simulink model "Wind_Turbine"  (Simulink 7.9)
settings: Solver=ode23t  StartTime=0.0  StopTime=80  MaxStep=0.01  RelTol=1e-5  AbsTol=1e-4
PreLoadFcn:
  | warning off Simulink:Commands:LoadMdlParameterizedLink
PostLoadFcn:
  | warning off Simulink:blocks:MatchingGotoNotFound
  | warning off Simulink:blocks:MatchingFromNotFound
  | warning('off','Simulink:SL_OutputNotConnected');
  | warning off Simulink:Engine:SaveWithParameterizedLinks_Warning
  | warning off Simulink:Engine:SaveWithDisabledLinks_Warning
  | warning('off','Simulink:fixpoint:fxpParameterPrecisionLoss');
  | warning off Simulink:blocks:DTConversionUncessary
  | warning off ne_sli:simulator:input:FilteredInputs
  | 
  | Setup_WT_Configurations
StartFcn:
  | tic
StopFcn:
  | Elapsed_Sim_Time = toc;
  | disp(['Elapsed time is ' num2str(Elapsed_Sim_Time)]);
undefined symbols (not defined in the file or in its folder): radps2rpm, WT_Params
libraries: powerlib x6, Wind_Lib x1, Blades_Lib x1, Generator_Lib x1, mblibv1 x1, Main_Controller_Lib x1, Nacelle_Lib x1, Pitch_Controller_Lib x1, Tower x1, Turbine_Input_Lib x1, Yaw_Controller_Lib x1
Description:
  | Copyright 2011 MathWorks, Inc.
settings Model: Creator=smiller  LastModifiedBy=smiller
settings SolverCC: MaxConsecutiveMinStep=5
settings DataIOCC: SaveFinalState=on
settings DebuggingCC: AlgebraicLoopMsg=error  ArtificialAlgebraicLoopMsg=none  SolverPrmCheckMsg=none  Int32ToFloatConvMsg=none  UnnecessaryDatatypeConvMsg=warning  FcnCallInpInsideContextMsg=Use local settings  StrictBusMsg=Warning
settings HardwareCC: TargetEndianess=LittleEndian  TargetHWDeviceType=MATLAB Host  ProdEqTarget=off
settings SFSimCC: SimParseCustomCode=off
settings RTWCC: ProcessScript=grt_make_rtw_hook
settings GRTTargetCC: CombineOutputUpdateFcns=off  GRTInterface=on
settings SimMechanicsCC: VisOnUpdateDiagram=on  VisDuringSimulation=on  FramesToBeSkipped=5  AnimationDelay=0  LastVizWinPosition=[16 233 560 424]  CamPosition=[-49.333;156.594;63.1057;]  CamTarget=[-1.98114;98.9678;-2.9194;]  CamUpVector=[0.335262;0.815674;-0.471461;]  CamHeight=16.8988  VisBackgroundColor=[0.678431;0.921569;1;]  DefaultBodyColor=[1;0;0;]
settings ConfigurationSet: Description=SimMechanics 2G

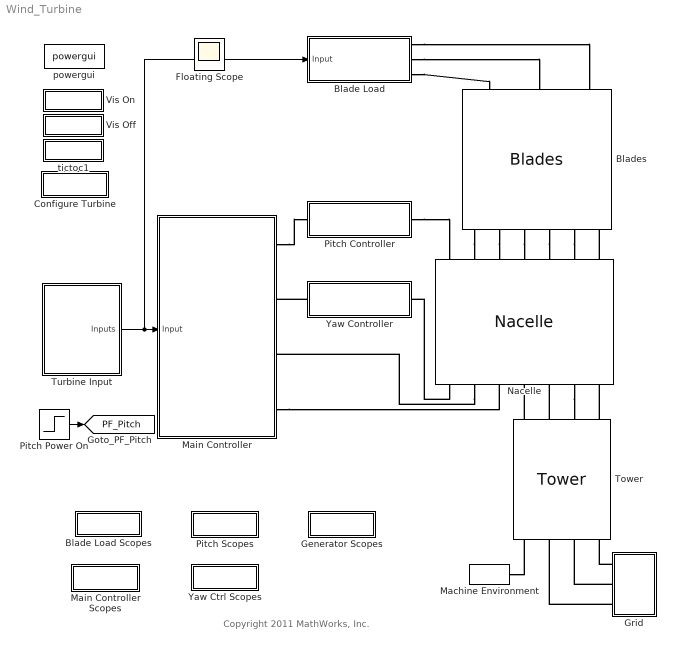
== system Wind_Turbine ==
  note: Copyright 2011 MathWorks, Inc.
  Blade Load : Subsystem  BlockChoice=Lift and Drag
      settings: AttributesFormatString=%<BlockChoice>  TemplateBlock=Wind_Lib/Blade Load  MemberBlocks=Lift and Drag,Lift and Drag (Simscape),Segments,Torque
  Blade Load Scopes : Subsystem  AncestorBlock=Wind_Lib/Blade Load Scopes
  Blades : Blades_Lib/Blades  RequirementInfo={'other' 'Wind_Turbine_Requirements.doc' '@overall_system' 'true' 'Blade Requirements ' ' ' } %GIDa_31eb547b_9de2_416c_ba1a_e68e51a35149  SystemSampleTime=-1
  Configure Turbine : Subsystem
  Generator Scopes : Subsystem  AncestorBlock=Generator_Lib/Generator Scopes
  Grid : Subsystem
  Machine Environment : mblibv1/Bodies/Machine Environment  PortType=env  PhysicalDomain=Mechanical  DialogTemplateClass=MECH.MachineEnvironment  SyncWhenCopied=off  Gravity=[0 -9.81 0]*0  GravityUnits=m/s^2  GravityAsSignal=off  Dimensionality=Auto-detect  AnalysisType=Forward dynamics  LinearAssemblyTolerance=1e-3  LinearAssemblyToleranceUnits=m  AngularAssemblyTolerance=1e-3  AngularAssemblyToleranceUnits=rad  ConstraintSolverType=Machine precision  ConstraintRelTolerance=1e-4  ConstraintAbsTolerance=1e-4  UseRobustSingularityHandling=off  RedundancyAnalysisToleranceType=Automatically select tolerance  RedundancyAnalysisTolerance=1e-14  StatePerturbationType=Fixed  PerturbationSize=1e-5  VisualizeMachine=on  BodyVisualizationType=Use model default body geometries  BodyColorSelMode=Use model default  DefaultBodyColor=[1 0 0]
  Main Controller : Subsystem  BlockChoice=Wind Input
      settings: AttributesFormatString=%<BlockChoice>  TemplateBlock=Main_Controller_Lib/Main Controller  MemberBlocks=Direct Input,Wind Input
  Main Controller Scopes : Subsystem  AncestorBlock=Main_Controller_Lib/Main Controller Scopes
  Nacelle : Nacelle_Lib/Nacelle  SystemSampleTime=-1
      link override Geartrain: BlockChoice=Empty
      link override Generator: BlockChoice=Simple
      link override Generator/Full/B_Gen/Model/VI/Ia: GotoTag=LibraryTag_Ia
      link override Generator/Full/B_Gen/Model/VI/Ib: GotoTag=LibraryTag_Ib
      link override Generator/Full/B_Gen/Model/VI/Ic: GotoTag=LibraryTag_Ic
      link override Generator/Full/B_Gen/Model/VI/Va: GotoTag=LibraryTag_Va
      link override Generator/Full/B_Gen/Model/VI/Vb: GotoTag=LibraryTag_Vb
      link override Generator/Full/B_Gen/Model/VI/Vc: GotoTag=LibraryTag_Vc
      link override Hub Axis: BlockChoice=Rotate
      link override Hub Axis/Rotate/3D-1D Mechanical Interface/Revolute - Rotational Interface/Joint Actuator: Primitive=R1  ActuationStyle=Force  TorqueUnits=N*m
      link override Hub Axis/Rotate/3D-1D Mechanical Interface/Revolute - Rotational Interface/Joint Sensor: Primitive=R1  Angle=off  ArcVelocity=on  ArcVelocityUnits=rad/s  ArcAcceleration=off  CoordPosition=off  Velocity=off  Acceleration=off  Quaternion=off  QuaternionDT=off  QuaternionDDT=off  Force=off  Torque=off  ReactionForce=off  ReactionMoment=off
      link override Hub Axis/Rotate/3D-1D Mechanical Interface/Revolute - Rotational Interface/PS-Simulink Converter: Unit=N*m
      link override Hub Axis/Rotate/3D-1D Mechanical Interface/Revolute - Rotational Interface/Simulink-PS Converter: Unit=rad/s
      link override Pitch System: BlockChoice=Ideal
      link override Yaw System: BlockChoice=Ideal Actuator
  Pitch Controller : Subsystem  BlockChoice=PI on AoA
      link override PI on AoA/Pitch Controller/Determine Pitch Command/Determine Angle of Attack if Pitch Angle Were 0/radps2mps: Gain=WT_Params.Blade.length
      settings: AttributesFormatString=%<BlockChoice>  TemplateBlock=Pitch_Controller_Lib/Pitch Controller  MemberBlocks=Inner Loop,PI on AoA
  Pitch Power On : Step  Time=20  Before=24  After=24  SampleTime=0
  Pitch Scopes : Subsystem  AncestorBlock=Pitch_Controller_Lib/Pitch Scopes
  Tower : Tower/Tower  RequirementInfo={'other' 'Wind_Turbine_Requirements.doc' '@Simulink_requirement_item_8' 'true' 'Tower Requirements' '' } %GIDa_4943b1c2_7ab1_472c_939d_e8be874b5a74  SystemSampleTime=-1
  Turbine Input : Subsystem  BlockChoice=Wind
      settings: AttributesFormatString=%<BlockChoice>  TemplateBlock=Turbine_Input_Lib/Turbine Input  MemberBlocks=Commands,Wind,Wind Cut Out,Wind High Speed,Wind Vary Speed
  Vis Off : Subsystem
      settings: OpenFcn=|
      | Temp_ENVHa= get_param(find_system(gcs,'LookUnderMasks','all','FollowLinks','on','ClassName','Environment'),'handle');
      | 
      | set_param(Temp_ENVHa{1},'VisualizeMachine','off');
      | 
      | set_param(gcs,'VisDuringSimulation','off')
      | set_param(gcs,'VisOnUpdateDiagram','off')
      mask Display: disp('Vis Off')
  Vis On : Subsystem
      settings: OpenFcn=|
      | Temp_ENVHa= get_param(find_system(gcs,'LookUnderMasks','all','FollowLinks','on','ClassName','Environment'),'handle');
      | 
      | set_param(Temp_ENVHa{1},'VisualizeMachine','on');
      | clear Temp_ENVHa;
      | set_param(gcs,'VisDuringSimulation','on')
      | set_param(gcs,'VisOnUpdateDiagram','on')
      mask Display: disp('Vis On')
  Yaw Controller : Subsystem  RequirementInfo={'other' 'Wind_Turbine_Requirements.doc' '@Simulink_requirement_item_7' 'true' 'Yaw Controller Requirements' '' } %GIDa_4e251ab5_598c_48b3_adbc_649df3f133e8  BlockChoice=Speed Limit
      settings: AttributesFormatString=%<BlockChoice>  TemplateBlock=Yaw_Controller_Lib/Yaw Controller  MemberBlocks=No Speed Limit,Speed Limit
  Yaw Ctrl Scopes : Subsystem  AncestorBlock=Yaw_Controller_Lib/Yaw Ctrl Scopes
  powergui : powerlib/powergui  SimulationMode=Phasor  SolverType=Tustin  SampleTime=1e-1  frequency=60  SPID=off  DisableSnubberDevices=off  DisableRonSwitches=off  DisableVfSwitches=off  SwTol=0  Interpol=off  DisplayEquations=off  FunctionMessages=off  frequencyindice=60  Pbase=100e6  ErrMax=1e-4  Iterations=50  UnitsV=kV  UnitsW=MW  echomessages=off  HookPort=off  EnableUseOfTLC=off  x0status=blocks  RestoreLinks=warning  ResistiveCurrentMeasurement=off  Frange=[0:2:500]  Ylog=off  Xlog=on  ShowGrid=off  save=off  variable=ZData  ZoomFFT=on  StartTime=0.0  cycles=1  DisplayStyle=1  fundamental=60  FreqAxis=off  MaxFrequency=1000  frequencyindicesteady=1  RmsSteady=1  display=off  Ts=0  methode=off
  tictoc1 : Subsystem
      settings: OpenFcn=open('Wind_Turbine_Demo_Script.html')
      mask Display: disp('Script')
  Floating Scope : Scope
      settings: Floating=on
  tag scope: PF_Pitch=global
  wires:
  Pitch Power On/1 -> [PF_Pitch]
  Turbine Input/1(Inputs) -> Blade Load/1(Input), Main Controller/1(Input)
  connections:
  Blades/LConn1 -- Nacelle/LConn2
  Pitch Controller/RConn1 -- Nacelle/LConn1
  Main Controller/RConn1 -- Pitch Controller/LConn1
  Tower/LConn2 -- Nacelle/RConn5
  Tower/LConn1 -- Nacelle/RConn4
  Machine Environment/RConn1 -- Tower/RConn1
  Blades/LConn5 -- Nacelle/LConn6
  Blades/LConn4 -- Nacelle/LConn5
  Blades/LConn3 -- Nacelle/LConn4
  Blades/LConn2 -- Nacelle/LConn3
  Nacelle/LConn7 -- Blades/LConn6
  Nacelle/RConn6 -- Tower/LConn3
  Tower/LConn4 -- Nacelle/RConn7
  Grid/RConn1 -- Tower/RConn4
  Grid/RConn2 -- Tower/RConn3
  Grid/RConn3 -- Tower/RConn2
  Yaw Controller/LConn1 -- Main Controller/RConn2
  Main Controller/RConn4 -- Nacelle/RConn3
  Nacelle/RConn2 -- Main Controller/RConn3
  Blade Load/RConn3 -- Blades/RConn1
  Blade Load/RConn2 -- Blades/RConn2
  Blade Load/RConn1 -- Blades/RConn3
  Nacelle/RConn1 -- Yaw Controller/RConn1

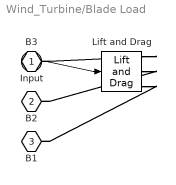
== system Wind_Turbine/Blade Load ==
  Input : Inport
  Lift and Drag : Wind_Lib/Lift and Drag  SystemSampleTime=-1
  B3 : PMIOPort  Port=1  Side=Right
  B2 : PMIOPort  Port=2  Side=Right
  B1 : PMIOPort  Port=3  Side=Right
  wires:
  Input/1 -> Lift and Drag/1
  connections:
  Lift and Drag/RConn1 -- B3/RConn1
  Lift and Drag/RConn2 -- B2/RConn1
  Lift and Drag/RConn3 -- B1/RConn1

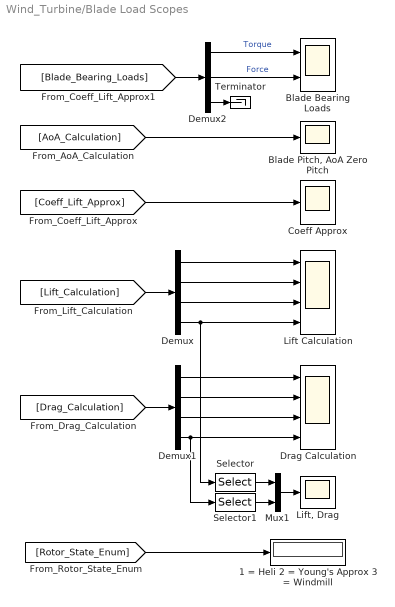
== system Wind_Turbine/Blade Load Scopes ==
  1 = Heli 2 = Young's Approx 3 = Windmill : Display
  Blade Bearing Loads : Scope  NumInputPorts=2
      settings: TimeRange=80  YMin=-2000000~-500000  YMax=4000000~500000  SaveName=ScopeData10
  "Blade Pitch, AoA Zero Pitch" : Scope
      settings: TimeRange=400  YMin=0  YMax=100  SaveName=ScopeData3
  Coeff Approx : Scope
      settings: TimeRange=400  YMin=-0.1139986551164904  YMax=0.01794057021302797  SaveName=ScopeData4
  Demux : Demux  Outputs=[1 3 3 3]
  Demux1 : Demux  Outputs=[1 3 3 3]
  Demux2 : Demux  Outputs=[3 3 12]
  Drag Calculation : Scope  NumInputPorts=4
      settings: TimeRange=400  YMin=-2000~-50~0~0  YMax=4000~100~6000~6000  SaveName=ScopeData5
  Lift Calculation : Scope  NumInputPorts=4
      settings: TimeRange=400  YMin=0~-50~-0.5~-50000  YMax=2000~100~1.5~100000  SaveName=ScopeData2
  "Lift, Drag" : Scope
      settings: TimeRange=160  YMin=-250.4351759669439  YMax=408.3026221352307
  Mux1 : Mux  Inputs=2
  Selector : Selector  InputPortWidth=3  IndexOptions=Index vector (dialog)  Indices=[1]  OutputSizes=1
  Selector1 : Selector  InputPortWidth=3  IndexOptions=Index vector (dialog)  Indices=[1 3]  OutputSizes=1
  Terminator : Terminator
  wires:
  Demux2/3 -> Terminator/1
  [Rotor_State_Enum] -> 1 = Heli 2 = Young's Approx 3 = Windmill/1
  Demux1/4 -> Drag Calculation/4, Selector1/1
  Demux1/3 -> Drag Calculation/3
  Demux1/2 -> Drag Calculation/2
  Demux1/1 -> Drag Calculation/1
  [Drag_Calculation] -> Demux1/1
  [Coeff_Lift_Approx] -> Coeff Approx/1
  Demux/4 -> Lift Calculation/4, Selector/1
  Demux/3 -> Lift Calculation/3
  Demux/2 -> Lift Calculation/2
  Demux/1 -> Lift Calculation/1
  [Lift_Calculation] -> Demux/1
  Mux1/1 -> "Lift, Drag"/1
  [AoA_Calculation] -> "Blade Pitch, AoA Zero Pitch"/1
  Selector/1 -> Mux1/1
  Selector1/1 -> Mux1/2
  [Blade_Bearing_Loads] -> Demux2/1
  Demux2/1 -> Blade Bearing Loads/1  "Torque"
  Demux2/2 -> Blade Bearing Loads/2  "Force"

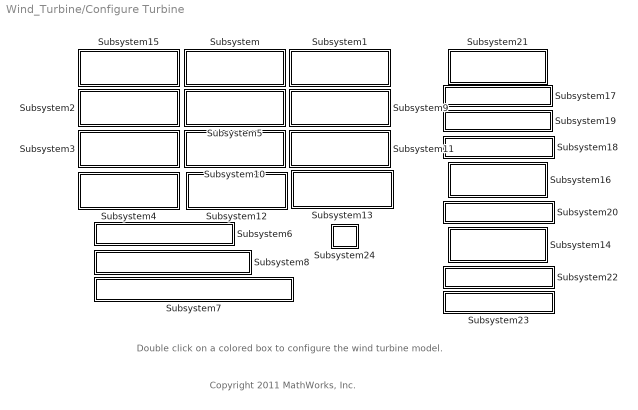
== system Wind_Turbine/Configure Turbine ==
  note: Copyright 2011 MathWorks, Inc.
  note: Double click on a colored box
      | to configure the wind turbine model.
  Subsystem : Subsystem
      settings: OpenFcn=Select_Turbine_Systems('I_Pitch Test', WT_Configs)
      mask Display: disp('Ideal\nPitch')
  Subsystem1 : Subsystem
      settings: OpenFcn=Select_Turbine_Systems('H_Pitch Test', WT_Configs)
      mask Display: disp('Hydraulic\nPitch')
  Subsystem10 : Subsystem
      settings: OpenFcn=Select_Turbine_Systems('I_Pitch IM_Yaw Test', WT_Configs)
      mask Display: disp('Ideal Pitch\nIdeal Motor Yaw')
  Subsystem11 : Subsystem
      settings: OpenFcn=Select_Turbine_Systems('H_Pitch IM_Yaw Test', WT_Configs)
      mask Display: disp('Hydraulic Pitch\nIdeal Motor Yaw')
  Subsystem12 : Subsystem
      settings: OpenFcn=Select_Turbine_Systems('I_Pitch S_Yaw Test', WT_Configs)
      mask Display: disp('Ideal Pitch\nServomotor Yaw')
  Subsystem13 : Subsystem
      settings: OpenFcn=Select_Turbine_Systems('H_Pitch S_Yaw Test', WT_Configs)
      mask Display: disp('Hydraulic Pitch\nServomotor Yaw')
  Subsystem14 : Subsystem
      settings: OpenFcn=Compare_Yaw_Actuators;
      mask Display: disp('Compare Yaw\nActuators')
  Subsystem15 : Subsystem
      mask Display: disp('TESTS')
  Subsystem16 : Subsystem
      settings: OpenFcn=Compare_Pitch_Actuators;
      mask Display: disp('Compare Pitch\nActuators')
  Subsystem17 : Subsystem
      settings: OpenFcn=Pitch_Actuation_Linkage
      mask Display: disp('Pitch Linkage')
  Subsystem18 : Subsystem
      settings: OpenFcn=Pitch_Actuation_Hydraulic_Testrig
      mask Display: disp('Hydr. Pitch Testrig')
  Subsystem19 : Subsystem
      settings: OpenFcn=Pitch_Control_Ideal_Testrig
      mask Display: disp('Ideal Pitch Testrig')
  Subsystem2 : Subsystem
      settings: OpenFcn=Select_Turbine_Systems('IA_Yaw Test', WT_Configs)
      mask Display: disp('Ideal Actuator\nYaw')
  Subsystem20 : Subsystem
      settings: OpenFcn=Yaw_Actuation_Testrig
      mask Display: disp('Yaw Testrig')
  Subsystem21 : Subsystem
      mask Display: disp('DEVELOP')
  Subsystem22 : Subsystem
      settings: OpenFcn=Generator_Testrig
      mask Display: disp('Generator Testrig')
  Subsystem23 : Subsystem
      settings: OpenFcn=Turbine_State_Machine_Testrig
      mask Display: disp('Supervisory Ctrl')
  Subsystem24 : Subsystem
      settings: OpenFcn=Select_Turbine_Systems('H_Pitch S_Yaw Ge Gn Lift_Drag', WT_Configs)
      mask Display: disp('C')
  Subsystem3 : Subsystem
      settings: OpenFcn=Select_Turbine_Systems('IM_Yaw Test', WT_Configs)
      mask Display: disp('Ideal Motor\nYaw')
  Subsystem4 : Subsystem
      settings: OpenFcn=Select_Turbine_Systems('S_Yaw Test', WT_Configs)
      mask Display: disp('Servomotor\nYaw')
  Subsystem5 : Subsystem
      settings: OpenFcn=Select_Turbine_Systems('I_Pitch IA_Yaw Test', WT_Configs)
      mask Display: disp('Ideal Pitch\nIdeal Act. Yaw')
  Subsystem6 : Subsystem
      settings: OpenFcn=Select_Turbine_Systems('I_Pitch IA_Yaw Lift_Drag', WT_Configs)
      mask Display: disp('I Pitch IA Yaw Lift Drag')
  Subsystem7 : Subsystem
      settings: OpenFcn=Select_Turbine_Systems('I_Pitch IA_Yaw Ge Gn Lift_Drag', WT_Configs)
      mask Display: disp('I_Pitch IA_Yaw Ge Gn Lift_Drag')
  Subsystem8 : Subsystem
      settings: OpenFcn=Select_Turbine_Systems('I_Pitch IA_Yaw Ge Lift_Drag', WT_Configs)
      mask Display: disp('I Pitch IA Yaw Ge Lift Drag')
  Subsystem9 : Subsystem
      settings: OpenFcn=Select_Turbine_Systems('H_Pitch IA_Yaw Test', WT_Configs)
      mask Display: disp('Hydraulic Pitch\nIdeal Act. Yaw')

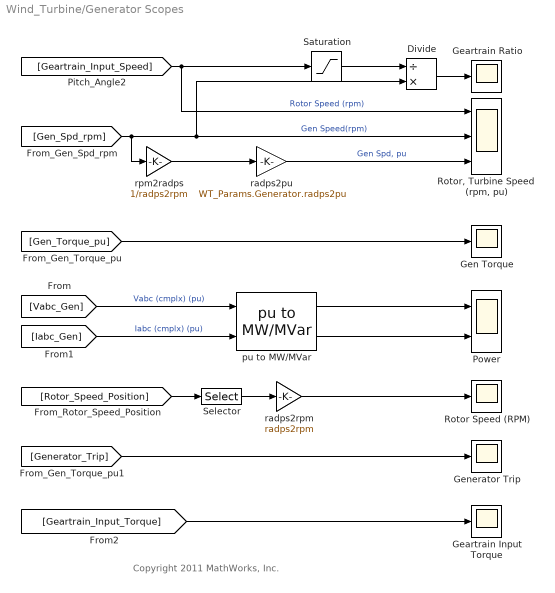
== system Wind_Turbine/Generator Scopes ==
  note: Copyright 2011 MathWorks, Inc.
  Divide : Product  Inputs=/*
  Geartrain Input Torque : Scope
      settings: TimeRange=80  YMin=-4000  YMax=-2250  SaveName=Geartrain_Input_Torque_DATA
  Geartrain Ratio : Scope
      settings: YMin=70  YMax=85  SaveName=ScopeData4
  Gen Torque : Scope
      settings: SaveName=ScopeData8
  Generator Trip : Scope
      settings: SaveName=Generator_Trip_DATA
  Power : Scope  NumInputPorts=2
      settings: TimeRange=80  YMin=-6000000~-6000000  YMax=4000000~0  SaveName=Generator_Power_DATA
  Rotor Speed (RPM) : Scope
      settings: TimeRange=80  YMin=0  YMax=15  SaveName=ScopeData6
  "Rotor, Turbine Speed  (rpm, pu)" : Scope  NumInputPorts=3
      settings: YMin=13.5~1100~0.9  YMax=15.5~1300~1.1  SaveName=Generator_Speed_DATA
  Saturation : Saturate  UpperLimit=inf  LowerLimit=eps
  Selector : Selector  InputPortWidth=2  IndexOptions=Index vector (dialog)  Indices=[2]  OutputSizes=1
  pu to MW/MVar : Generator_Lib/Generator Scopes/pu to MW//MVar
  radps2pu : Gain  Gain=WT_Params.Generator.radps2pu
  radps2rpm : Gain  Gain=radps2rpm
  rpm2radps : Gain  Gain=1/radps2rpm
  wires:
  [Generator_Trip] -> Generator Trip/1
  pu to MW/MVar/2 -> Power/2
  pu to MW/MVar/1 -> Power/1
  [Gen_Torque_pu] -> Gen Torque/1
  [Iabc_Gen] -> pu to MW/MVar/2  "Iabc (cmplx) (pu)"
  [Vabc_Gen] -> pu to MW/MVar/1  "Vabc (cmplx) (pu)"
  [Geartrain_Input_Speed] -> "Rotor, Turbine Speed  (rpm, pu)"/1, Saturation/1  "Rotor Speed (rpm)"
  radps2pu/1 -> "Rotor, Turbine Speed  (rpm, pu)"/3  "Gen Spd, pu"
  rpm2radps/1 -> radps2pu/1
  Divide/1 -> Geartrain Ratio/1
  [Gen_Spd_rpm] -> "Rotor, Turbine Speed  (rpm, pu)"/2, Divide/2, rpm2radps/1  "Gen Speed(rpm)"
  [Rotor_Speed_Position] -> Selector/1
  Selector/1 -> radps2rpm/1
  radps2rpm/1 -> Rotor Speed (RPM)/1
  Saturation/1 -> Divide/1
  [Geartrain_Input_Torque] -> Geartrain Input Torque/1

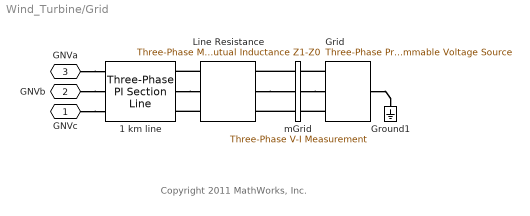
== system Wind_Turbine/Grid ==
  note: Copyright 2011 MathWorks, Inc.
  "1 km line " : powerlib/Elements/Three-Phase PI Section Line  LConnTagsString=a|b|c  RConnTagsString=A|B|C  Frequency=WT_Params.Grid.frequency  Resistances=[0.1153 0.413]  Inductances=[1.05e-3 3.32e-3]  Capacitances=[11.33e-009 5.01e-009]  Length=1
  Grid : powerlib/Electrical Sources/Three-Phase Programmable Voltage Source  PositiveSequence=[WT_Params.Grid.voltage 0 WT_Params.Grid.frequency]  VariationEntity=None  VariationType=Table of time-amplitude pairs  VariationTypeAlt=Step  VariationStep=-0.15  VariationRate=10  VariationMagnitude=0.3  VariationFrequency=2  VariationTiming=[5 5.5]  VariationPhaseA=off  Amplitudes="[1.0  0.5  1.0 ]"  TimeValues="[0  10  10.1]"  HarmonicGeneration=off  HarmonicA=[1 -0.1 0 1]  HarmonicB=[2 0.15 35 2]  Timing="[5  5.5]"  BusType=swing  Pref=0  Qref=0  Qmin=-inf  Qmax=inf
  Ground1 : powerlib/Elements/Ground  LConnTagsString=a
  Line Resistance : powerlib/Elements/Three-Phase Mutual Inductance Z1-Z0  LConnTagsString=a|b|c  RConnTagsString=A|B|C  PositiveSequence="[0.1  1.0/(2*pi*60)]*WT_Params.Grid.voltage^2/2500e6"  ZeroSequence="[0.3  3.0/(2*pi*60)]*WT_Params.Grid.voltage^2/2500e6"
  mGrid : powerlib/Measurements/Three-Phase V-I Measurement  VoltageMeasurement=phase-to-ground  SetLabelV=on  LabelV=VmGrid  Vpu=on  VpuLL=off  CurrentMeasurement=no  SetLabelI=on  LabelI=ImGrid  Ipu=off  Pbase=1.5e6/0.9  Vbase=25e3  OutputType=Magnitude  PhasorSimulation=on  PSBequivalent=0
  GNVc : PMIOPort  Port=1  Side=Right
  GNVb : PMIOPort  Port=2  Side=Right
  GNVa : PMIOPort  Port=3  Side=Right
  connections:
  Line Resistance/RConn1 -- "1 km line "/LConn1
  "1 km line "/LConn2 -- Line Resistance/RConn2
  Line Resistance/RConn3 -- "1 km line "/LConn3
  Grid/LConn1 -- Ground1/LConn1
  Grid/RConn1 -- mGrid/LConn1
  mGrid/LConn2 -- Grid/RConn2
  Grid/RConn3 -- mGrid/LConn3
  mGrid/RConn1 -- Line Resistance/LConn1
  Line Resistance/LConn2 -- mGrid/RConn2
  mGrid/RConn3 -- Line Resistance/LConn3
  GNVa/RConn1 -- "1 km line "/RConn1
  GNVb/RConn1 -- "1 km line "/RConn2
  GNVc/RConn1 -- "1 km line "/RConn3

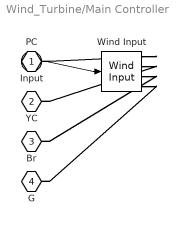
== system Wind_Turbine/Main Controller ==
  Input : Inport
  Wind Input : Main_Controller_Lib/Wind Input  SystemSampleTime=-1
  PC : PMIOPort  Port=1  Side=Right
  YC : PMIOPort  Port=2  Side=Right
  Br : PMIOPort  Port=3  Side=Right
  G : PMIOPort  Port=4  Side=Right
  wires:
  Input/1 -> Wind Input/1
  connections:
  Wind Input/RConn1 -- PC/RConn1
  Wind Input/RConn2 -- YC/RConn1
  Wind Input/RConn3 -- Br/RConn1
  Wind Input/RConn4 -- G/RConn1

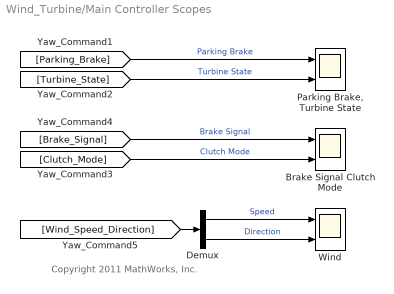
== system Wind_Turbine/Main Controller Scopes ==
  note: Copyright 2011 MathWorks, Inc.
  Brake Signal Clutch Mode : Scope  NumInputPorts=2
      settings: TimeRange=80  YMin=-1~1  YMax=1~3  SaveName=ScopeData9
  Demux : Demux  Outputs=2
  "Parking Brake, Turbine State" : Scope  NumInputPorts=2
      settings: TimeRange=80  YMin=0~0  YMax=1~3  SaveName=ScopeData7
  Wind : Scope  NumInputPorts=2
      settings: TimeRange=80  YMin=0~-5  YMax=20~5  SaveName=Wind_Turbine_Wind_DATA
  wires:
  [Parking_Brake] -> "Parking Brake, Turbine State"/1  "Parking Brake"
  [Turbine_State] -> "Parking Brake, Turbine State"/2  "Turbine State"
  [Brake_Signal] -> Brake Signal Clutch Mode/1  "Brake Signal"
  [Clutch_Mode] -> Brake Signal Clutch Mode/2  "Clutch Mode"
  [Wind_Speed_Direction] -> Demux/1
  Demux/1 -> Wind/1  "Speed"
  Demux/2 -> Wind/2  "Direction"

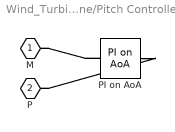
== system Wind_Turbine/Pitch Controller ==
  PI on AoA : Pitch_Controller_Lib/PI on AoA  SystemSampleTime=-1
  M : PMIOPort  Port=1  Side=Left
  P : PMIOPort  Port=2  Side=Right
  connections:
  PI on AoA/LConn1 -- M/RConn1
  PI on AoA/RConn1 -- P/RConn1

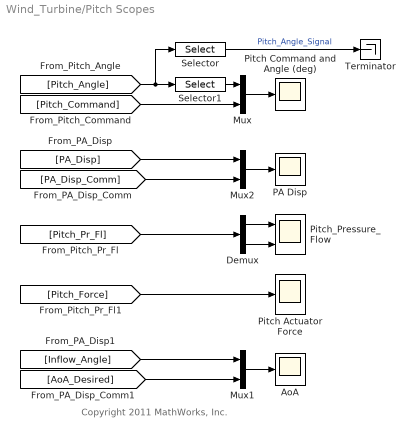
== system Wind_Turbine/Pitch Scopes ==
  note: Copyright 2011 MathWorks, Inc.
  AoA : Scope
      settings: TimeRange=10  YMin=-1.6  YMax=-0.9  SaveName=ScopeData2
  Demux : Demux  Outputs=[2 1]
  Mux : Mux  Inputs=2
  Mux1 : Mux  Inputs=2
  Mux2 : Mux  Inputs=2
  PA Disp : Scope
      settings: TimeRange=10  YMin=-1.6  YMax=-0.9
  Pitch Actuator Force : Scope
      settings: TimeRange=80  YMin=-78125  YMax=84375  SaveName=Pitch_Actuator_Force_DATA
  Pitch Command and Angle (deg) : Scope
      settings: TimeRange=80  YMin=-20  YMax=80  SaveName=Blade_Pitch_DATA
  Pitch_Pressure_Flow : Scope  NumInputPorts=2
      settings: YMin=-5~-5  YMax=20~5  SaveName=ScopeData3
  Selector : Selector  InputPortWidth=3  IndexOptions=Index vector (dialog)  Indices=[1 ]  OutputSizes=1
  Selector1 : Selector  InputPortWidth=3  IndexOptions=Index vector (dialog)  Indices=[1 ]  OutputSizes=1
  Terminator : Terminator
  wires:
  [Pitch_Force] -> Pitch Actuator Force/1
  Selector/1 -> Terminator/1  "Pitch_Angle_Signal"
  Demux/2 -> Pitch_Pressure_Flow/2
  Demux/1 -> Pitch_Pressure_Flow/1
  [Pitch_Pr_Fl] -> Demux/1
  [PA_Disp_Comm] -> Mux2/2
  Mux2/1 -> PA Disp/1
  [PA_Disp] -> Mux2/1
  Mux/1 -> Pitch Command and Angle (deg)/1
  [Pitch_Command] -> Mux/2
  [Pitch_Angle] -> Selector/1, Selector1/1
  [AoA_Desired] -> Mux1/2
  Mux1/1 -> AoA/1
  [Inflow_Angle] -> Mux1/1
  Selector1/1 -> Mux/1

== system Wind_Turbine/Turbine Input ==
  Wind : Turbine_Input_Lib/Wind  SystemSampleTime=-1
  Inputs : Outport
  wires:
  Wind/1 -> Inputs/1

== system Wind_Turbine/Vis Off ==

== system Wind_Turbine/Vis On ==

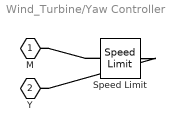
== system Wind_Turbine/Yaw Controller ==
  Speed Limit : Yaw_Controller_Lib/Speed Limit  SystemSampleTime=-1
  M : PMIOPort  Port=1  Side=Left
  Y : PMIOPort  Port=2  Side=Right
  connections:
  Speed Limit/LConn1 -- M/RConn1
  Speed Limit/RConn1 -- Y/RConn1

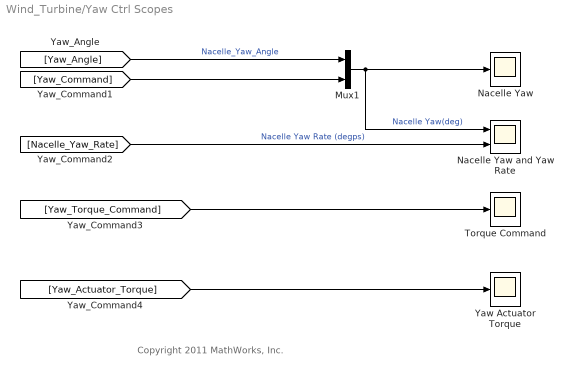
== system Wind_Turbine/Yaw Ctrl Scopes ==
  note: Copyright 2011 MathWorks, Inc.
  Mux1 : Mux  Inputs=2
  Nacelle Yaw : Scope
      settings: TimeRange=80  SaveName=Nacelle_Yaw_DATA
  Nacelle Yaw and Yaw Rate : Scope  NumInputPorts=2
      settings: TimeRange=80  YMin=-5~-0.8  YMax=5~0.6000000000000001  SaveName=ScopeData7
  Torque Command : Scope
      settings: TimeRange=3.951473136915078
  Yaw Actuator Torque : Scope
      settings: TimeRange=80  YMin=-517076.6058045388  YMax=509833.5093808146  SaveName=Yaw_Actuator_Torque_DATA
  wires:
  [Nacelle_Yaw_Rate] -> Nacelle Yaw and Yaw Rate/2  "Nacelle Yaw Rate (degps)"
  Mux1/1 -> Nacelle Yaw/1, Nacelle Yaw and Yaw Rate/1  "Nacelle Yaw(deg)"
  [Yaw_Command] -> Mux1/2
  [Yaw_Angle] -> Mux1/1  "Nacelle_Yaw_Angle"
  [Yaw_Torque_Command] -> Torque Command/1
  [Yaw_Actuator_Torque] -> Yaw Actuator Torque/1

== system Wind_Turbine/tictoc1 ==

== system Wind_Turbine/Configure Turbine/Subsystem ==

== system Wind_Turbine/Configure Turbine/Subsystem1 ==

== system Wind_Turbine/Configure Turbine/Subsystem10 ==

== system Wind_Turbine/Configure Turbine/Subsystem11 ==

== system Wind_Turbine/Configure Turbine/Subsystem12 ==

== system Wind_Turbine/Configure Turbine/Subsystem13 ==

== system Wind_Turbine/Configure Turbine/Subsystem14 ==

== system Wind_Turbine/Configure Turbine/Subsystem15 ==

== system Wind_Turbine/Configure Turbine/Subsystem16 ==

== system Wind_Turbine/Configure Turbine/Subsystem17 ==

== system Wind_Turbine/Configure Turbine/Subsystem18 ==

== system Wind_Turbine/Configure Turbine/Subsystem19 ==

== system Wind_Turbine/Configure Turbine/Subsystem2 ==

== system Wind_Turbine/Configure Turbine/Subsystem20 ==

== system Wind_Turbine/Configure Turbine/Subsystem21 ==

== system Wind_Turbine/Configure Turbine/Subsystem22 ==

== system Wind_Turbine/Configure Turbine/Subsystem23 ==

== system Wind_Turbine/Configure Turbine/Subsystem24 ==

== system Wind_Turbine/Configure Turbine/Subsystem3 ==

== system Wind_Turbine/Configure Turbine/Subsystem4 ==

== system Wind_Turbine/Configure Turbine/Subsystem5 ==

== system Wind_Turbine/Configure Turbine/Subsystem6 ==

== system Wind_Turbine/Configure Turbine/Subsystem7 ==

== system Wind_Turbine/Configure Turbine/Subsystem8 ==

== system Wind_Turbine/Configure Turbine/Subsystem9 ==
